simulink model "RCS"  (R2023b)
settings: Solver=FixedStepAuto  StartTime=0.0  StopTime=tf  FixedStep=step_modelo  RelTol=1e-3
values from neighbouring files (symbols this model uses):
  step_modelo = 0.1    [ControleOrbital_Entradas.m]    (also in GuiamentoDinamicaCinematicaOrbital_Entradas.m)
undefined symbols (not defined in the file or in its folder): actuator, actuator_nonlin, Fn, mib, rb, tc, Td, Tpulse
settings Model: PacingRate=0.100000  Creator=rodri  LastModifiedBy=rodri

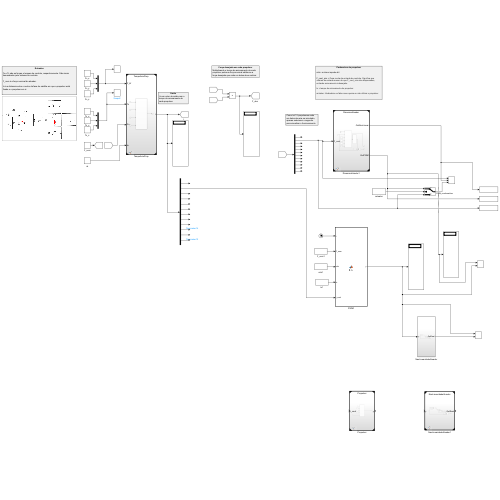
[thumbnail: Simulink's stored preview of the top-level diagram]
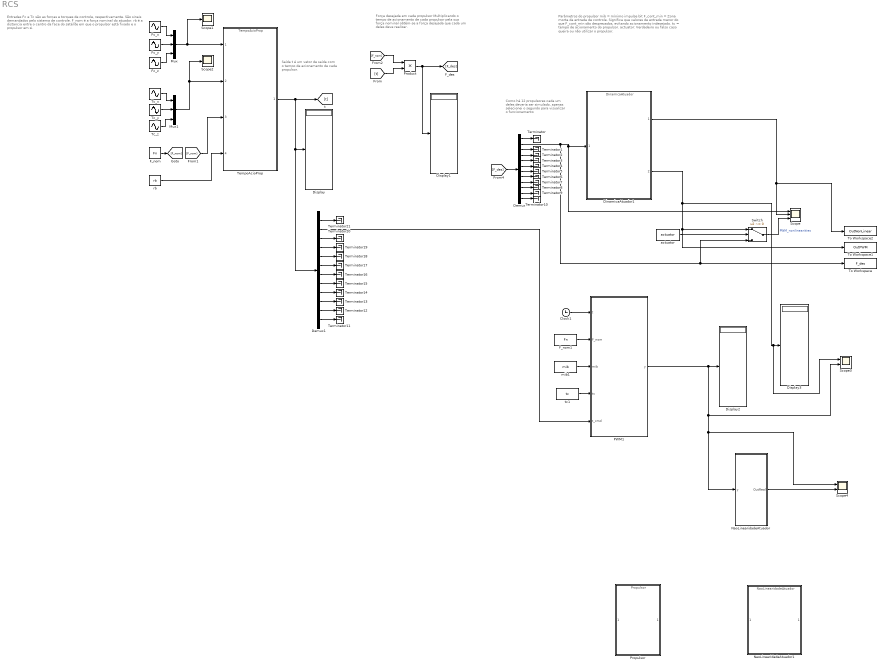
== system RCS ==
  note: Como há 12 propulsores cada um deles deveria ser simulado, apenas selecionei o segundo para visualizar o funcionamento
  note: Entradas
      |
      | Fc e Tc são as forças e torques de controle, respectivamente. São sinais demandados pelo sistema de controle.
      |
      | F_nom é a força nominal do atuador.
      |
      | rb é a distancia entre o centro da face do satélite em que o propulsor está fixado e o propulsor em si.
  note: Saída
      | t é um vetor de saída com o tempo de acionamento de cada propulsor.
  note: Parâmetros do propulsor
      |
      | mib = mínimo impulse bit
      |
      | F_cont_min = Zona morta da entrada de controle. Significa que valores de entrada menor do que F_cont_min são desprezados, evitando acionamento indesejado.
      |
      | tc = tempo de acionamento do propulsor.
      |
      | actuator: Verdadeiro ou falso caso queira ou não utilizar o propulsor.
  note: Força desejada em cada propulsor
      | Multiplicando o tempo de acionamento de cada propulsor pela sua força nominal obtêm-se a força desejada que cada um deles deve realizar.
  Clock1 : Clock
  Demux : Demux  Outputs=12
  Demux1 : Demux  Outputs=12
  DinamicaAtuador1 : ModelReference  ModelNameDialog=DinamicaAtuador  ModelReferenceVersion=2.4
  Display{,1..3} (4 alike) : Display
  F_nom : Constant  Value=Fn  SampleTime=step_modelo
  F_nom1 : Constant  Value=Fn  SampleTime=-1
  Fc_x : Sin  SampleTime=step_modelo
  Fc_y : Sin  Amplitude=0  SampleTime=step_modelo
  Fc_z : Sin  Amplitude=0  SampleTime=step_modelo
  Mux : Mux  Inputs=3
  Mux1 : Mux  Inputs=3
  NaoLinearidadeAtuador : Subsystem
  NaoLinearidadeAtuador1 : ModelReference  ModelNameDialog=NaoLinearidadeAtuador  ModelReferenceVersion=1.14
  PWM1 : MATLAB Function  TreatAsAtomicUnit=on
  Product : Product
  Propulsor : ModelReference  ModelNameDialog=Propulsor  ModelReferenceVersion=1.13
  Scope : Scope  NumInputPorts=3
  Scope1 : Scope
  Scope2 : Scope
  Scope3 : Scope  NumInputPorts=2
  Scope4 : Scope  NumInputPorts=2
  Switch : Switch  Criteria=u2 ~= 0  SaturateOnIntegerOverflow=off  InputSameDT=off
  Tc_x : Sin  Amplitude=0.2  SampleTime=step_modelo
  Tc_y : Sin  Amplitude=0  SampleTime=step_modelo
  Tc_z : Sin  Amplitude=0  SampleTime=step_modelo
  TempoAcioProp : ModelReference  ModelNameDialog=TempoAcioProp.slx  ModelReferenceVersion=2.1
  Terminator{,1..21} (22 alike) : Terminator
  To Workspace : ToWorkspace  VariableName=F_des  SaveFormat=Timeseries  SampleTime=-1
  To Workspace1 : ToWorkspace  VariableName=OutPWM  SaveFormat=Timeseries  SampleTime=-1
  To Workspace2 : ToWorkspace  VariableName=OutNonLinear  SaveFormat=Timeseries  SampleTime=-1
  actuator : Constant  Value=actuator  OutDataTypeStr=boolean  SampleTime=-1
  mib1 : Constant  Value=mib  SampleTime=-1
  rb : Constant  Value=rb  SampleTime=step_modelo
  tc1 : Constant  Value=tc  SampleTime=-1
  wires:
  Product/1 -> [F_des], Display1/1
  Demux/1 -> Terminator/1
  Demux/12 -> Terminator10/1
  actuator/1 -> Switch/2
  Demux/7 -> Terminator5/1
  Demux/11 -> Terminator9/1
  [F_des] -> Demux/1
  Demux/6 -> Terminator4/1
  Tc_y/1 -> Mux1/2
  Demux/5 -> Terminator3/1
  [F_nom] -> TempoAcioProp/3
  Demux/4 -> Terminator2/1
  Demux/10 -> Terminator8/1
  Switch/1 -> Scope/3  "PWM_nonlinearities"
  Demux/2 -> Scope/1, DinamicaAtuador1/1, To Workspace/1, Switch/3
  Demux/9 -> Terminator7/1
  F_nom/1 -> [F_nom]
  Tc_z/1 -> Mux1/3
  Tc_x/1 -> Mux1/1
  Demux/3 -> Terminator1/1
  [F_nom] -> Product/1
  Fc_y/1 -> Mux/2
  rb/1 -> TempoAcioProp/4
  TempoAcioProp/1 -> [t], Demux1/1, Display/1
  [t] -> Product/2
  Demux/8 -> Terminator6/1
  Fc_z/1 -> Mux/3
  Fc_x/1 -> Mux/1
  Mux/1 -> Scope1/1, TempoAcioProp/1
  DinamicaAtuador1/2 -> Scope3/1, Display3/1, Switch/1, To Workspace1/1
  DinamicaAtuador1/1 -> Scope/2, To Workspace2/1
  Mux1/1 -> Scope2/1, TempoAcioProp/2
  tc1/1 -> PWM1/4(tc)
  Clock1/1 -> PWM1/1(t)
  mib1/1 -> PWM1/3(mib)
  F_nom1/1 -> PWM1/2(F_nom)
  Demux1/2 -> PWM1/5(t_cmd)
  Demux1/12 -> Terminator11/1
  Demux1/11 -> Terminator12/1
  Demux1/10 -> Terminator13/1
  Demux1/9 -> Terminator14/1
  Demux1/8 -> Terminator15/1
  Demux1/7 -> Terminator16/1
  Demux1/6 -> Terminator17/1
  Demux1/5 -> Terminator18/1
  Demux1/4 -> Terminator19/1
  Demux1/3 -> Terminator20/1
  Demux1/1 -> Terminator21/1
  PWM1/1(y) -> Scope4/1, NaoLinearidadeAtuador/1(y), Scope3/2, Display2/1
  NaoLinearidadeAtuador/1(OutReal) -> Scope4/2

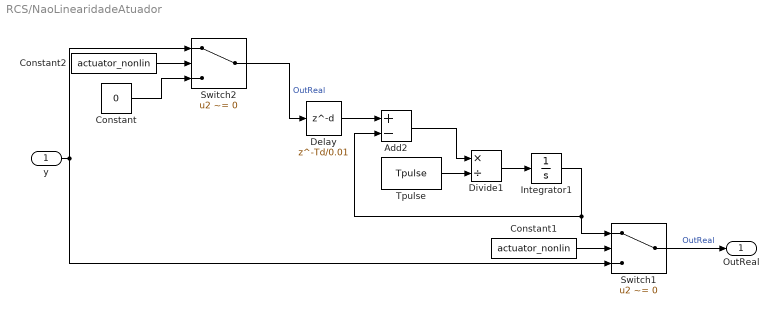
== system RCS/NaoLinearidadeAtuador ==
  y : Inport
  Add2 : Sum  Inputs=+-
  Constant : Constant  Value=0
  Constant1 : Constant  Value=actuator_nonlin  OutDataTypeStr=boolean  SampleTime=-1
  Constant2 : Constant  Value=actuator_nonlin  OutDataTypeStr=boolean  SampleTime=-1
  Delay : Delay  DelayLength=Td/0.01  InitialCondition=0
  Divide1 : Product  Inputs=*/
  Integrator1 : Integrator
  Switch1 : Switch  Criteria=u2 ~= 0  SaturateOnIntegerOverflow=off  InputSameDT=off
  Switch2 : Switch  Criteria=u2 ~= 0  SaturateOnIntegerOverflow=off  InputSameDT=off
  Tpulse : Constant  Value=Tpulse  SampleTime=-1
  OutReal : Outport
  wires:
  Switch1/1 -> OutReal/1  "OutReal"
  Constant1/1 -> Switch1/2
  Integrator1/1 -> Switch1/1, Add2/2
  Tpulse/1 -> Divide1/2
  Delay/1 -> Add2/1
  y/1 -> Switch2/1, Switch1/3
  Add2/1 -> Divide1/1
  Divide1/1 -> Integrator1/1
  Constant2/1 -> Switch2/2
  Switch2/1 -> Delay/1  "OutReal"
  Constant/1 -> Switch2/3

== matlab function RCS/PWM1 ==
  data: t input; F_nom input; mib input; tc input; y output; t_cmd input
function y  = fcn(t,F_nom,mib,tc,t_cmd)

control_cycle = 1/tc;

if t_cmd >0 && t_cmd <= mib
    t_cmd = mib;
    pulse_cmd = 100*t_cmd/control_cycle; %porcentagem de atuação (%)
    duty=pulse_cmd;
else
    pulse_cmd = 100*t_cmd/control_cycle; %porcentagem de atuação (%)
    duty=pulse_cmd;
end

y = F_nom*square(2*pi*control_cycle.*t,duty);
if y <= 0
    y = 0;
end
